simulink model "Observers"  (R2021a)
settings: Solver=VariableStepAuto  StartTime=0.0  StopTime=10.0  RelTol=1e-3
values from neighbouring files (symbols this model uses):
  bEh = 2*(bhd + bhm*ih^2)/rhd^2    (= 31004.4444444)    [Data.m]
  bEtd = (btd + btm*it^2)/rtd^2    (= 21607.2)    [Data.m]
  bhb = 1.0e8    (= 100000000)    [Data.m]
  bhEb = 2.2e9    (= 2200000000)    [Data.m]
  btb = 5.0e6    (= 5000000)    [Data.m]
  g = 9.80665    [Data.m]
  ih = 22    [Data.m]
  it = 30    [Data.m]
  MEh = 2*(Jhd_hEb + Jhm_hb * ih^2)/rhd^2    (= 65137.7777778)    [Data.m]
  MEtd = (Jtd + Jtm_tb*it^2)/rtd^2    (= 30000)    [Data.m]
  Ms = 15000    [Data.m]
  rhd = 0.75    [Data.m]
  rtd = 0.5    [Data.m]
  Thb_max = 5.0e4    (= 50000)    [Data.m]
  ThEb_max = 1.1e6    (= 1100000)    [Data.m]
  Ttb_max = 5.0e3    (= 5000)    [Data.m]
settings Model: Creator=jpss8  LastModifiedBy=jpss8

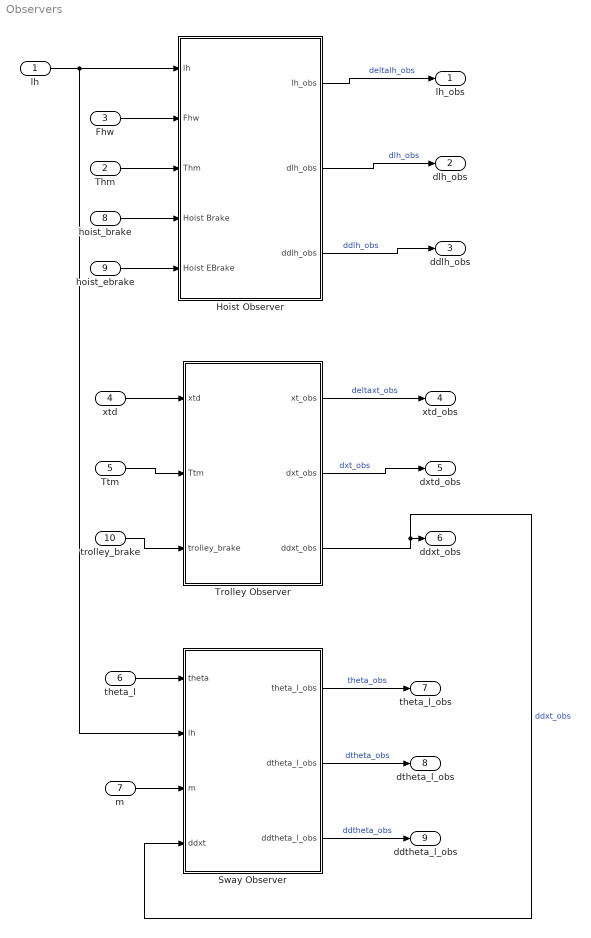
== system Observers ==
  lh : Inport
  Thm : Inport  Port=2
  Fhw : Inport  Port=3
  xtd : Inport  Port=4
  Ttm : Inport  Port=5
  theta_l : Inport  Port=6
  m : Inport  Port=7
  hoist_brake : Inport  Port=8
  hoist_ebrake : Inport  Port=9
  trolley_brake : Inport  Port=10
  Hoist Observer : Subsystem
  Sway Observer : Subsystem
  Trolley Observer : Subsystem
  lh_obs : Outport
  dlh_obs : Outport  Port=2
  ddlh_obs : Outport  Port=3
  xtd_obs : Outport  Port=4
  dxtd_obs : Outport  Port=5
  ddxt_obs : Outport  Port=6
  theta_l_obs : Outport  Port=7
  dtheta_l_obs : Outport  Port=8
  ddtheta_l_obs : Outport  Port=9
  wires:
  Trolley Observer/1(xt_obs) -> xtd_obs/1  "deltaxt_obs"
  Fhw/1 -> Hoist Observer/2(Fhw)
  m/1 -> Sway Observer/3(m)
  Trolley Observer/2(dxt_obs) -> dxtd_obs/1  "dxt_obs"
  Hoist Observer/1(lh_obs) -> lh_obs/1  "deltalh_obs"
  theta_l/1 -> Sway Observer/1(theta)
  Hoist Observer/3(ddlh_obs) -> ddlh_obs/1  "ddlh_obs"
  lh/1 -> Sway Observer/2(lh), Hoist Observer/1(lh)
  Hoist Observer/2(dlh_obs) -> dlh_obs/1  "dlh_obs"
  xtd/1 -> Trolley Observer/1(xtd)
  Trolley Observer/3(ddxt_obs) -> Sway Observer/4(ddxt), ddxt_obs/1  "ddxt_obs"
  Sway Observer/1(theta_l_obs) -> theta_l_obs/1  "theta_obs"
  Sway Observer/2(dtheta_l_obs) -> dtheta_l_obs/1  "dtheta_obs"
  Sway Observer/3(ddtheta_l_obs) -> ddtheta_l_obs/1  "ddtheta_obs"
  Thm/1 -> Hoist Observer/3(Thm)
  Ttm/1 -> Trolley Observer/2(Ttm)
  hoist_brake/1 -> Hoist Observer/4(Hoist Brake)
  hoist_ebrake/1 -> Hoist Observer/5(Hoist EBrake)
  trolley_brake/1 -> Trolley Observer/3(trolley_brake)

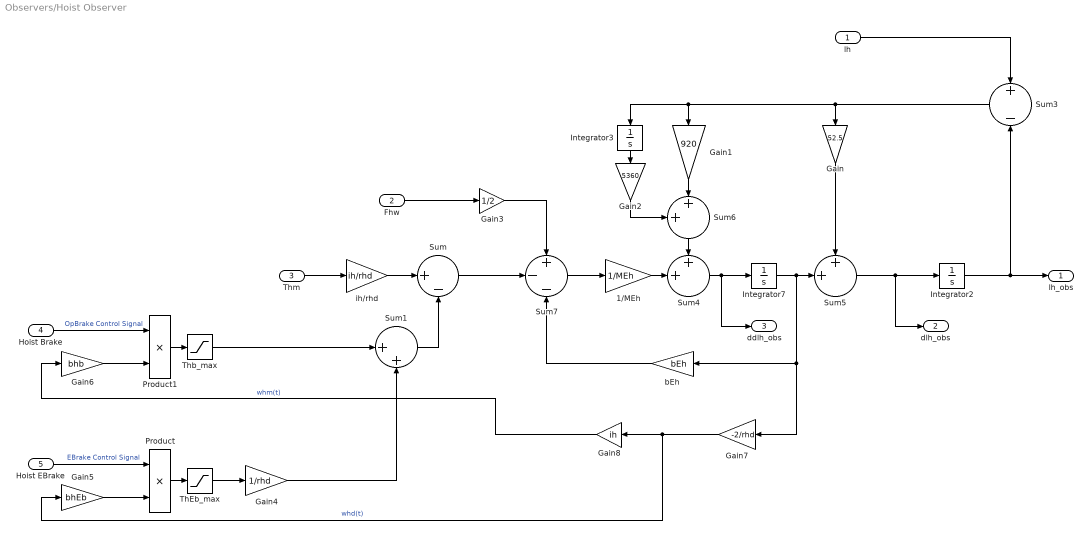
== system Observers/Hoist Observer ==
  lh : Inport
  Fhw : Inport  Port=2
  Thm : Inport  Port=3
  Hoist Brake : Inport  Port=4
  Hoist EBrake : Inport  Port=5
  1/MEh : Gain  Gain=1/MEh
  Gain : Gain  Gain=52.5
  Gain1 : Gain  Gain=920
  Gain2 : Gain  Gain=5360
  Gain3 : Gain  Gain=1/2
  Gain4 : Gain  Gain=1/rhd
  Gain5 : Gain  Gain=bhEb
  Gain6 : Gain  Gain=bhb
  Gain7 : Gain  Gain=-2/rhd
  Gain8 : Gain  Gain=ih
  Integrator2 : Integrator
  Integrator3 : Integrator
  Integrator7 : Integrator
  Product : Product
  Product1 : Product
  Sum : Sum  Inputs=|+-
  Sum1 : Sum  Inputs=|++
  Sum3 : Sum  Inputs=+|-
  Sum4 : Sum  Inputs=++|
  Sum5 : Sum  Inputs=++|
  Sum6 : Sum  Inputs=++|
  Sum7 : Sum  Inputs=+--
  ThEb_max : Saturate  UpperLimit=ThEb_max  LowerLimit=-ThEb_max
  Thb_max : Saturate  UpperLimit=Thb_max  LowerLimit=-Thb_max
  bEh : Gain  Gain=bEh
  ih/rhd : Gain  Gain=ih/rhd
  lh_obs : Outport
  dlh_obs : Outport  Port=2
  ddlh_obs : Outport  Port=3
  wires:
  Sum5/1 -> dlh_obs/1, Integrator2/1
  lh/1 -> Sum3/1
  Gain1/1 -> Sum6/2
  Gain3/1 -> Sum7/1
  Integrator3/1 -> Gain2/1
  bEh/1 -> Sum7/3
  Sum3/1 -> Gain/1, Integrator3/1, Gain1/1
  ih/rhd/1 -> Sum/1
  Sum7/1 -> 1/MEh/1
  Sum4/1 -> ddlh_obs/1, Integrator7/1
  Gain/1 -> Sum5/1
  Integrator2/1 -> Sum3/2, lh_obs/1
  Sum6/1 -> Sum4/1
  Integrator7/1 -> Gain7/1, bEh/1, Sum5/2
  1/MEh/1 -> Sum4/2
  Thm/1 -> ih/rhd/1
  Fhw/1 -> Gain3/1
  Gain2/1 -> Sum6/1
  Product/1 -> ThEb_max/1
  Gain5/1 -> Product/2
  Hoist Brake/1 -> Product1/1  "OpBrake Control Signal"
  Gain7/1 -> Gain5/1, Gain8/1  "whd(t)"
  Product1/1 -> Thb_max/1
  Gain6/1 -> Product1/2
  ThEb_max/1 -> Gain4/1
  Gain4/1 -> Sum1/2
  Hoist EBrake/1 -> Product/1  "EBrake Control Signal"
  Thb_max/1 -> Sum1/1
  Sum/1 -> Sum7/2
  Sum1/1 -> Sum/2
  Gain8/1 -> Gain6/1  "whm(t)"

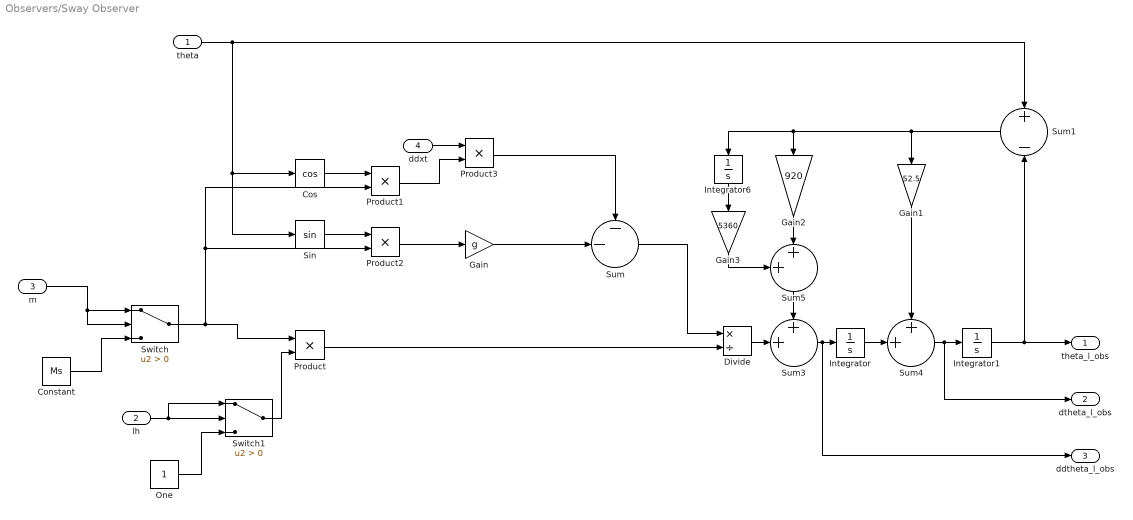
== system Observers/Sway Observer ==
  theta : Inport
  lh : Inport  Port=2
  m : Inport  Port=3
  ddxt : Inport  Port=4
  Constant : Constant  Value=Ms
  Cos : Trigonometry  Operator=cos
  Divide : Product  Inputs=*/
  Gain : Gain  Gain=g
  Gain1 : Gain  Gain=52.5
  Gain2 : Gain  Gain=920
  Gain3 : Gain  Gain=5360
  Integrator : Integrator
  Integrator1 : Integrator
  Integrator6 : Integrator
  One : Constant  OutDataTypeStr=Inherit: Inherit via back propagation
  Product{,1..3} (4 alike) : Product
  Sin : Trigonometry
  Sum : Sum  Inputs=--|
  Sum1 : Sum  Inputs=+|-
  Sum3 : Sum  Inputs=++|
  Sum4 : Sum  Inputs=++|
  Sum5 : Sum  Inputs=++|
  Switch : Switch  Criteria=u2 > Threshold
  Switch1 : Switch  Criteria=u2 > Threshold
  theta_l_obs : Outport
  dtheta_l_obs : Outport  Port=2
  ddtheta_l_obs : Outport  Port=3
  wires:
  Product/1 -> Divide/2
  theta/1 -> Sin/1, Cos/1, Sum1/1
  lh/1 -> Switch1/1, Switch1/2
  Divide/1 -> Sum3/2
  Product3/1 -> Sum/1
  Cos/1 -> Product1/1
  Sin/1 -> Product2/1
  Product2/1 -> Gain/1
  Gain/1 -> Sum/2
  Product1/1 -> Product3/2
  ddxt/1 -> Product3/1
  Sum/1 -> Divide/1
  Integrator1/1 -> theta_l_obs/1, Sum1/2
  Sum1/1 -> Gain1/1, Gain2/1, Integrator6/1
  Gain2/1 -> Sum5/2
  Gain3/1 -> Sum5/1
  Sum3/1 -> ddtheta_l_obs/1, Integrator/1
  Sum4/1 -> dtheta_l_obs/1, Integrator1/1
  Sum5/1 -> Sum3/1
  Gain1/1 -> Sum4/1
  Integrator/1 -> Sum4/2
  m/1 -> Switch/2, Switch/1
  Switch/1 -> Product/1, Product1/2, Product2/2
  Constant/1 -> Switch/3
  Integrator6/1 -> Gain3/1
  Switch1/1 -> Product/2
  One/1 -> Switch1/3

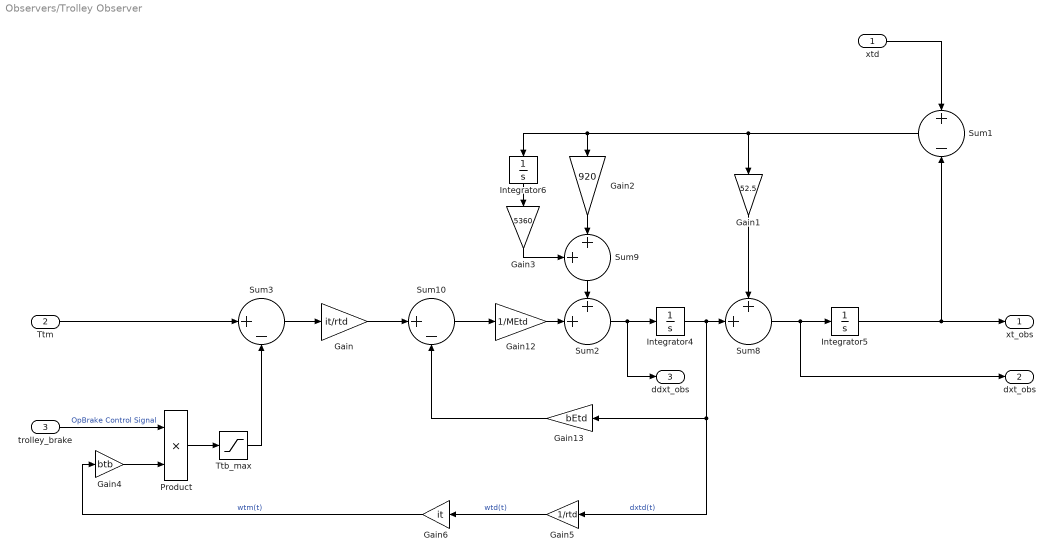
== system Observers/Trolley Observer ==
  xtd : Inport
  Ttm : Inport  Port=2
  trolley_brake : Inport  Port=3
  Gain : Gain  Gain=it/rtd
  Gain1 : Gain  Gain=52.5
  Gain12 : Gain  Gain=1/MEtd
  Gain13 : Gain  Gain=bEtd
  Gain2 : Gain  Gain=920
  Gain3 : Gain  Gain=5360
  Gain4 : Gain  Gain=btb
  Gain5 : Gain  Gain=1/rtd
  Gain6 : Gain  Gain=it
  Integrator4 : Integrator
  Integrator5 : Integrator
  Integrator6 : Integrator
  Product : Product
  Sum1 : Sum  Inputs=+|-
  Sum10 : Sum  Inputs=|+-
  Sum2 : Sum  Inputs=++|
  Sum3 : Sum  Inputs=|+-
  Sum8 : Sum  Inputs=++|
  Sum9 : Sum  Inputs=++|
  Ttb_max : Saturate  UpperLimit=Ttb_max  LowerLimit=-Ttb_max
  xt_obs : Outport
  dxt_obs : Outport  Port=2
  ddxt_obs : Outport  Port=3
  wires:
  Sum2/1 -> ddxt_obs/1, Integrator4/1
  Sum8/1 -> Integrator5/1, dxt_obs/1
  Sum1/1 -> Gain1/1, Gain2/1, Integrator6/1
  Integrator5/1 -> Sum1/2, xt_obs/1
  xtd/1 -> Sum1/1
  Gain12/1 -> Sum2/2
  Gain2/1 -> Sum9/2
  Gain/1 -> Sum10/1
  Gain13/1 -> Sum10/2
  Sum10/1 -> Gain12/1
  Gain3/1 -> Sum9/1
  Sum9/1 -> Sum2/1
  Ttm/1 -> Sum3/1
  Integrator6/1 -> Gain3/1
  Gain1/1 -> Sum8/1
  Product/1 -> Ttb_max/1
  trolley_brake/1 -> Product/1  "OpBrake Control Signal"
  Gain4/1 -> Product/2
  Sum3/1 -> Gain/1
  Ttb_max/1 -> Sum3/2
  Gain5/1 -> Gain6/1  "wtd(t)"
  Gain6/1 -> Gain4/1  "wtm(t)"
  Integrator4/1 -> Sum8/2, Gain13/1, Gain5/1  "dxtd(t)"
